simulink model "kilogram_TO_pound"  (R2021a)
settings: Solver=VariableStepAuto  StartTime=0.0  StopTime=10.0  RelTol=1e-3
settings Model: Creator=MAC  LastModifiedBy=MAC

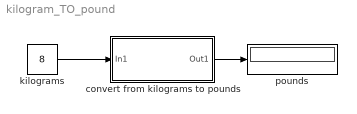
== system kilogram_TO_pound ==
  convert from kilograms to pounds : Subsystem
  kilograms : Constant  Value=8
  pounds : Display
  wires:
  kilograms/1 -> convert from kilograms to pounds/1(In1)
  convert from kilograms to pounds/1(Out1) -> pounds/1

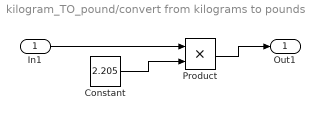
== system kilogram_TO_pound/convert from kilograms to pounds ==
  In1 : Inport
  Constant : Constant  Value=2.205
  Product : Product
  Out1 : Outport
  wires:
  In1/1 -> Product/1
  Product/1 -> Out1/1
  Constant/1 -> Product/2
